simulink model "attitude_controller_rev"  (R2021b)
settings: Solver=FixedStepDiscrete  StartTime=0.0  StopTime=25  FixedStep=1/40  RelTol=1e-3
PreLoadFcn:
  | load('var_roll.mat')
model workspace (MAT data in the model file):
  cmdLim = Simulink.Parameter
  cmdLim.Value = 15
  cmdLim.Description = 'This is the limit for controlling the maximum surface command angle.'
  cmdLim.DataType = 'auto'
  cmdLim.Min = 0
  cmdLim.Max = 90
  cmdLim.DocUnits = 'deg'
  cmdLim.Complexity = 'real'
  cmdLim.Dimensions = [1 1]
  dispGain = Simulink.Parameter
  dispGain.Value = 0.75
  dispGain.Description = 'This is the gain applied to the displacement error.'
  dispGain.DataType = 'auto'
  dispGain.Min = 0
  dispGain.DocUnits = 'deg/sec/deg'
  dispGain.Complexity = 'real'
  dispGain.Dimensions = [1 1]
  dispLim = Simulink.Parameter
  dispLim.Value = 30
  dispLim.Description = 'This is the limit for controlling the maximum commanded angle.'
  dispLim.DataType = 'auto'
  dispLim.Min = 0
  dispLim.Max = 180
  dispLim.DocUnits = 'deg'
  dispLim.Complexity = 'real'
  dispLim.Dimensions = [1 1]
  intGain = Simulink.Parameter
  intGain.Value = 0.5
  intGain.Description = 'This is the gain applied to the integral error.'
  intGain.DataType = 'auto'
  intGain.Min = 0
  intGain.DocUnits = 'deg/sec/deg/sec'
  intGain.Complexity = 'real'
  intGain.Dimensions = [1 1]
  intLim = Simulink.Parameter
  intLim.Value = 5
  intLim.Description = 'This is the limit for controlling the maximum commanded angle.'
  intLim.DataType = 'auto'
  intLim.Min = 0
  intLim.Max = 90
  intLim.DocUnits = 'deg'
  intLim.Complexity = 'real'
  intLim.Dimensions = [1 1]
  rateGain = Simulink.Parameter
  rateGain.Value = 2
  rateGain.Description = 'This is the gain applied to the rate error.'
  rateGain.DataType = 'auto'
  rateGain.Min = 0
  rateGain.DocUnits = 'deg/deg/sec'
  rateGain.Complexity = 'real'
  rateGain.Dimensions = [1 1]
  rateLim = Simulink.Parameter
  rateLim.Value = 6
  rateLim.Description = 'This is the limit for controlling the maximum commanded angle.'
  rateLim.DataType = 'auto'
  rateLim.Min = 0
  rateLim.Max = 180
  rateLim.DocUnits = 'deg/sec'
  rateLim.Complexity = 'real'
  rateLim.Dimensions = [1 1]
libraries: simulink x1, AP_Lib_rev x1
settings Model: RequirementInfo={} %GIDa_eb906a4c_0ec7_43a1_b5c3_86a9990349a4  FPTRunName=FPA_Reference  reqMgrSettings="100 S'doors','misc'{{S'surrogatepath','savemodel','savesurrogate','doorsLinks2sl','slLinks2Doors','detaillevel','surrogateId','synctime'{{T\"/Autopilot Project/attitude_controller\",M[1],M[1],M[1],M[1],M[1],T\"00000040\",T\"\"}},S'mode','pathStorage'{{T\"generic\",T\"modelRelative\"}}}}"  ParameterArgumentNames=dispGain,dispLim,rateGain,rateLim,intGain,intLim,cmdLim  Creator=bpotter  LastModifiedBy=achan260
settings SolverCC: AlgebraicLoopSolver=TrustRegion
settings DataIOCC: ExternalInput=attitudeIn  SaveFormat=StructureWithTime  SaveOutput=off  DSMLogging=off  SaveTime=off  ReturnWorkspaceOutputs=off  SignalLoggingName=attitude_Controller_logsout
settings OptimizationCC: BlockReduction=off  DefaultParameterBehavior=Inlined  InlineInvariantSignals=on  ExpressionDepthLimit=2147483647  EfficientFloat2IntCast=on  EfficientMapNaN2IntZero=off  LifeSpan=inf  MaxStackSize=inf  EfficientTunableParamExpr=on
settings DebuggingCC: SignalInfNanChecking=error  SignalRangeChecking=error  ReadBeforeWriteMsg=EnableAllAsError  WriteAfterWriteMsg=EnableAllAsError  WriteAfterReadMsg=EnableAllAsError  AlgebraicLoopMsg=error  ArtificialAlgebraicLoopMsg=error  SaveWithDisabledLinksMsg=error  SaveWithParameterizedLinksMsg=error  CheckExecutionContextPreStartOutputMsg=on  BlockPriorityViolationMsg=error  MaxConsecutiveZCsMsg=warning  SolverPrmCheckMsg=error  InheritedTsInSrcMsg=error  SingleTaskRateTransMsg=error  TasksWithSamePriorityMsg=error  SigSpecEnsureSampleTimeMsg=error  CheckMatrixSingularityMsg=error  IntegerOverflowMsg=error  ParameterUnderflowMsg=error  ParameterPrecisionLossMsg=error  ParameterTunabilityLossMsg=error  UnderSpecifiedDataTypeMsg=error  UnnecessaryDatatypeConvMsg=warning  VectorMatrixConversionMsg=error  SignalLabelMismatchMsg=error  UnconnectedInputMsg=error  UnconnectedOutputMsg=error  UnconnectedLineMsg=error  SFcnCompatibilityMsg=error  UniqueDataStoreMsg=error  BusObjectLabelMismatch=error  RootOutportRequireBusObject=error  AssertControl=DisableAll  ModelReferenceIOMsg=error  ModelReferenceIOMismatchMessage=error  UnknownTsInhSupMsg=error  ModelReferenceDataLoggingMessage=error  ModelReferenceExtraNoncontSigs=none  StateNameClashWarn=warning  StrictBusMsg=ErrorOnBusTreatedAsVector  NonBusSignalsTreatedAsBus=error  SFUnexpectedBacktrackingDiag=warning  SFNoUnconditionalDefaultTransitionDiag=warning  SFMachineParentedDataDiag=warning  IntegerSaturationMsg=error  ArithmeticOperatorsInVariantConditions=warning
settings HardwareCC: ProdBitPerPointer=32  ProdBitPerSizeT=32  ProdBitPerPtrDiffT=32  ProdLargestAtomicFloat=None  ProdEndianess=BigEndian  ProdWordSize=32  ProdHWDeviceType=32-bit Embedded Processor  TargetHWDeviceType=32-bit Generic
settings ModelReferenceCC: PropagateSignalLabelsOutOfModel=off
settings SFSimCC: SimUseLocalCustomCode=off  MATLABDynamicMemAlloc=off  CustomCodeUndefinedFunction=UseInterfaceOnly
settings RTWCC: Description=Embedded Coder  SystemTargetFile=ert.tlc  TemplateMakefile=ert_default_tmf  GenerateReport=on  RTWVerbose=off  RTWUseLocalCustomCode=off  IncludeHyperlinkInReport=on  LaunchReport=on  PortableWordSizes=on  GenerateTraceInfo=on  GenerateTraceReport=on  GenerateTraceReportSl=on  GenerateTraceReportSf=on  GenerateTraceReportEml=on
settings CodeAppCC: ForceParamTrailComments=on  IgnoreCustomStorageClasses=off  MaxIdLength=63  MangleLength=4  CustomSymbolStrType=$N$R$M  StateflowObjectComments=on  InternalIdentifier=Classic  ReqsInCode=on
settings ERTTargetCC: UtilityFuncGeneration=Shared location  MultiwordLength=2048  IncludeMdlTerminateFcn=off  SuppressErrorStatus=on  SupportAbsoluteTime=off  SupportNonFinite=off  SupportComplex=off  ParenthesesLevel=Maximum  InlinedParameterPlacement=NonHierarchical  MultiInstanceErrorCode=None  ERTCustomFileTemplate=example_file_process.tlc  PreserveExpressionOrder=on  PreserveIfCondition=on  ConvertIfToSwitch=off  SuppressUnreachableDefaultCases=off
settings ConfigComp: CovSaveName=attitude_controller_covdata  CovMetricSettings=dcmtrzoiwe  CovHTMLOptions=-sRT=1 -aTS=1 -bRG=1 -bTC=1 -hTR=1 -nFC=0 -scm=1 -bcm=1 -xEv=0  CovSaveCumulativeToWorkspaceVar=on  CovCumulativeVarName=attitude_controller_covCumulativeData  CovCumulativeReport=on  CovReportOnPause=off  CovExternalEMLEnable=off

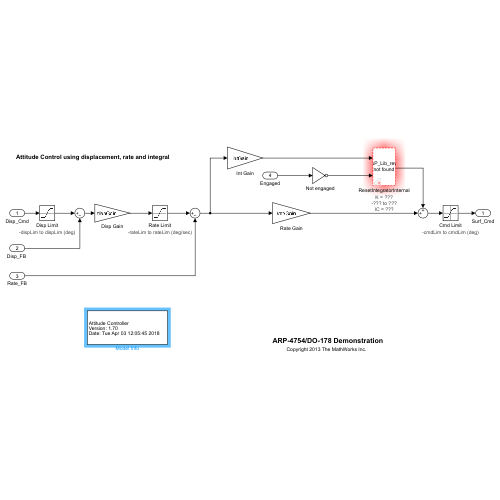
[thumbnail: Simulink's stored preview of the top-level diagram]
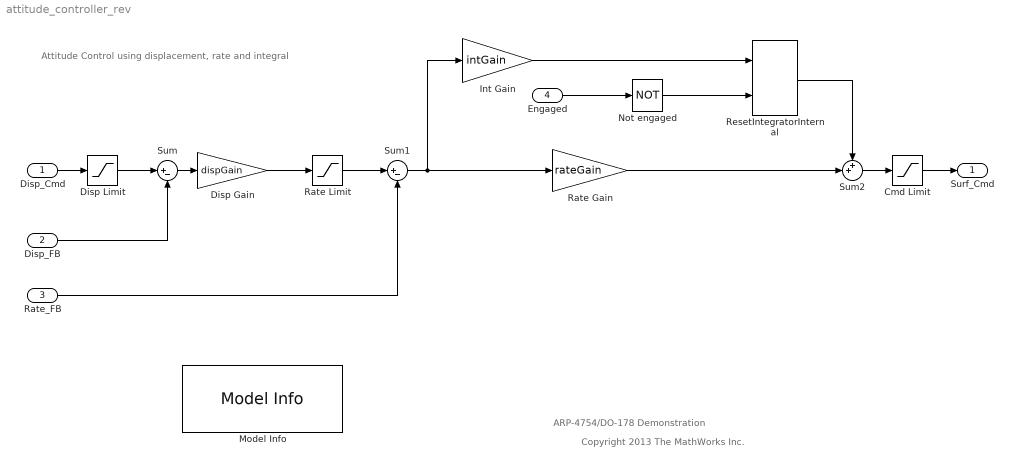
== system attitude_controller_rev ==
  note: Attitude Control using displacement, rate and integral
  note: Copyright 2013 The MathWorks Inc.
  note: ARP-4754/DO-178 Demonstration
  Disp_Cmd : Inport  RequirementInfo={} %GIDa_1f6c7271_93c3_4f3b_ad46_40b2620097e5  OutDataTypeStr=double  PortDimensions=1  SampleTime=1/40
  "Disp_FB " : Inport  RequirementInfo={} %GIDa_a4c10b54_79b2_494f_9fbb_11aba459525d  Port=2  OutDataTypeStr=double  PortDimensions=1  SampleTime=1/40
  Rate_FB : Inport  RequirementInfo={} %GIDa_8a5ee350_5b96_4034_aa7b_307fc7a5da71  Port=3  OutDataTypeStr=double  PortDimensions=1  SampleTime=1/40
  Engaged : Inport  RequirementInfo={} %GIDa_99509e30_ac8c_4d41_82c3_48695d972b31  Port=4  OutDataTypeStr=boolean  PortDimensions=1  SampleTime=1/40
  Cmd Limit : Saturate  RequirementInfo={} %GIDa_ec5fb8d1_63e1_4cbf_bd50_e97ea1f3a86f  UpperLimit=cmdLim  LowerLimit=-cmdLim
      settings: AttributesFormatString=%<LowerLimit> to %<UpperLimit> (deg)
  Disp Gain : Gain  RequirementInfo={} %GIDa_4fcfcfe9_3275_4fa9_885f_cf306a71b936  Gain=dispGain
  Disp Limit : Saturate  RequirementInfo={} %GIDa_7b92da27_c5ec_485b_a9fa_f73a890a94ea  UpperLimit=dispLim  LowerLimit=-dispLim
      settings: AttributesFormatString=%<LowerLimit> to %<UpperLimit> (deg)
  Int Gain : Gain  RequirementInfo={} %GIDa_beea6fba_2894_42ca_8163_07bc86b02f8e  Gain=intGain
  Model Info : simulink/Model-Wide Utilities/Model Info  Frame=on  DisplayStringWithTags=|  HorizontalTextAlignment=Left  LeftAlignmentValue=0.02
      | Attitude Controller
      | Version: %<ModelVersion>
      | Date: %<LastModificationDate>
  Not engaged : Logic  RequirementInfo={} %GIDa_955db51c_db14_42aa_b67d_de05482530f8  Operator=NOT  IconShape=distinctive  AllPortsSameDT=off  OutDataTypeStr=boolean
  Rate Gain : Gain  RequirementInfo={} %GIDa_4fe20f02_adbd_4ca0_a7f6_fed161d48486  Gain=rateGain
  Rate Limit : Saturate  RequirementInfo={} %GIDa_6ae337a4_f989_4d2e_9517_e05a98139e9b  UpperLimit=rateLim  LowerLimit=-rateLim
      settings: AttributesFormatString=%<LowerLimit> to %<UpperLimit> (deg/sec)
  ResetIntegratorInternal : AP_Lib_rev/ResetIntegratorInternal  K=1.0  Ts=1/40  IC=0  UL=intLim
      settings: AttributesFormatString=K = %<K>\n-%<UL> to %<UL>\nIC = %<IC>
  Sum : Sum  RequirementInfo={} %GIDa_cf5e480a_5b22_4e1a_9467_aeba7515f114  Inputs=|+-
  Sum1 : Sum  RequirementInfo={} %GIDa_37a43aee_ff03_4021_a10a_39656d6638a3  Inputs=|+-
  Sum2 : Sum  RequirementInfo={} %GIDa_fadb0a26_a1fd_480b_9f5d_0b7f45001c5e  Inputs=++|
  Surf_Cmd : Outport  RequirementInfo={} %GIDa_99d2b8ce_ab27_4685_9887_a082a0698432  OutDataTypeStr=double  PortDimensions=1  SampleTime=1/40
  wires:
  Disp_Cmd/1 -> Disp Limit/1
  "Disp_FB "/1 -> Sum/2
  Rate_FB/1 -> Sum1/2
  Sum1/1 -> Rate Gain/1, Int Gain/1
  Disp Gain/1 -> Rate Limit/1
  Sum/1 -> Disp Gain/1
  Disp Limit/1 -> Sum/1
  Rate Limit/1 -> Sum1/1
  Cmd Limit/1 -> Surf_Cmd/1
  Rate Gain/1 -> Sum2/2
  Sum2/1 -> Cmd Limit/1
  Engaged/1 -> Not engaged/1
  ResetIntegratorInternal/1 -> Sum2/1
  Int Gain/1 -> ResetIntegratorInternal/1
  Not engaged/1 -> ResetIntegratorInternal/2
